simulink model "submarine"  (R2014b)
settings: Solver=ode45  StartTime=0.0  StopTime=100.0  RelTol=1e-3
settings Model: Creator=Yuantao  LastModifiedBy=Yuantao

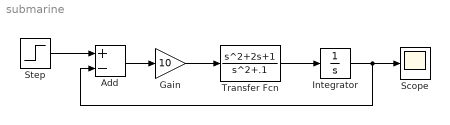
== system submarine ==
  Add : Sum  Inputs=+-
  Gain : Gain  Gain=10
  Integrator : Integrator
  Scope : Scope
  Step : Step  After=-50  SampleTime=0
  Transfer Fcn : TransferFcn  Numerator=[1 2 1]  Denominator=[1 0 .1]
  wires:
  Add/1 -> Gain/1
  Step/1 -> Add/1
  Gain/1 -> Transfer Fcn/1
  Transfer Fcn/1 -> Integrator/1
  Integrator/1 -> Add/2, Scope/1
